simulink model "problem8"  (R2020b)
settings: Solver=VariableStepAuto  StartTime=0.0  StopTime=10.0  RelTol=1e-3
settings Model: Creator=Lenovo  LastModifiedBy=Lenovo

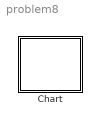
== system problem8 ==
  Chart : Stateflow chart  TreatAsAtomicUnit=on

== stateflow chart problem8/Chart ==
  state Lift [parallel]
    settings: executionOrder=2
    state floor0
      entry:temp=0;
    state floor1
      entry:temp=temp+1;
    state floor2
      entry:temp=temp+1;
    state floor3
      entry:temp=temp+1;
    state floor4
      entry:temp=temp+1;
      exit:temp=0;
    (default) -> floor0
    floor0 -> floor1 : [input1 >temp]
    floor1 -> floor0 [order 1] : [input1 == 0]
    floor1 -> floor2 [order 2] : [input1>temp]
    floor2 -> floor1 [order 1] : [input1<=1]
    floor2 -> floor3 [order 2] : [input1>temp]
    floor3 -> floor2 [order 1] : [input1<=2]
    floor3 -> floor4 [order 2] : [input1>temp]
    floor4 -> floor3 : [input1<=3]
  state Start [parallel]
    input1=call;
    settings: executionOrder=1
  data: x function_output; temp local; input1 local
  function x= call:
    | function x= call
    | x=randi([0,4]);
    | end
